simulink model "LATC_Test_Calc"  (R2021b)
settings: Solver=FixedStepDiscrete  StartTime=0.0  StopTime=inf  FixedStep=0.01  RelTol=1e-3
values from neighbouring files (symbols this model uses):
  P_Global_CharSpd_ms : value not decoded    [PubParsGlobal.sldd]
  P_Global_SteeringAngleRatio : value not decoded    [PubParsGlobal.sldd]
  P_Global_WheelBase_m : value not decoded    [PubParsGlobal.sldd]
  P_LCS_A0_Dis_BP : value not decoded    [SubMdlDD_LATC.sldd]
  P_LCS_A2_Curve_BP : value not decoded    [SubMdlDD_LATC.sldd]
  P_LCS_A2_LatAcc_BP : value not decoded    [SubMdlDD_LATC.sldd]
  P_LCS_A2_Pretime = 0.075    [SubMdlDD_LATC.sldd]
  P_LCS_A2S_FliterTime = 0.5    [SubMdlDD_LATC.sldd]
  P_LCS_AngleFilterTime = 0.1    [SubMdlDD_LATC.sldd]
  P_LCS_AngleSlope_AES_Active = 0.4 0.4 0.4 0.35 0.35 0.35 0.35 0.35 0.35 0.3 0.3 0.3 0.3 0.3 0.3 0.3 0.3 0.3 0.3 0.4 0.4 0.4 0.35 0.35 0.35 0.35 0.35 0.35 0.3 0.3 0.3 0.3 0.3 0.3 0.3 0.3 0.3 0.3 0.4 0.4 0.4 0.35 0.35 0.35 0.35 0.35 0.35 0.3 0.3 0.3 0.3 0.3 0.3 0.3 0.3 0.3 0.3 0.4 0.4 0.4 0.35 0.35 0.35 0.35 0.35 0.35 0.3 0.3 0.3 0.3 0.3 0.3 0.3 0.3 0.3 0.3 0.4 0.4 0.4 0.35 0.35 0.35 0.35 0.35 0.35 0.3 0.3 0.3 0.3 0.3 0.3 0.3 0.    [SubMdlDD_LATC.sldd]
  P_LCS_AngleSlope_ESS_Add = 1.0 1.0 1.0 1.0 2.0 2.0 2.0 7.0 7.0 7.0 7.0 7.0 7.0 7.0 7.0 7.0 7.0 7.0 7.0 1.0 1.0 1.0 1.0 2.0 2.0 2.0 7.0 7.0 7.0 7.0 7.0 7.0 7.0 7.0 7.0 7.0 7.0 7.0 1.0 1.0 1.0 1.0 2.0 2.0 2.0 7.0 7.0 7.0 7.0 7.0 7.0 7.0 7.0 7.0 7.0 7.0 7.0 1.0 1.0 1.0 1.0 2.0 2.0 2.0 7.0 7.0 7.0 7.0 7.0 7.0 7.0 7.0 7.0 7.0 7.0 7.0 1.0 1.0 1.0 1.0 7.5 7.5 7.5 7.5 7.5 7.5 7.5 7.5 7.5 7.5 7.5 8.0 8.0 8.0 8.0 1.0 1.0 1.0 1.0 7.5    [SubMdlDD_LATC.sldd]
  P_LCS_AngleSlope_LC_Eco = 0.4 0.4 0.4 0.35 0.35 0.35 0.35 0.35 0.35 0.3 0.3 0.3 0.3 0.3 0.3 0.3 0.3 0.3 0.3 0.4 0.4 0.4 0.35 0.35 0.35 0.35 0.35 0.35 0.3 0.3 0.3 0.3 0.3 0.3 0.3 0.3 0.3 0.3 0.4 0.4 0.4 0.35 0.35 0.35 0.35 0.35 0.35 0.3 0.3 0.3 0.3 0.3 0.3 0.3 0.3 0.3 0.3 0.4 0.4 0.4 0.35 0.35 0.35 0.35 0.35 0.35 0.3 0.3 0.3 0.3 0.3 0.3 0.3 0.3 0.3 0.3 0.4 0.4 0.4 0.35 0.35 0.35 0.35 0.35 0.35 0.3 0.3 0.3 0.3 0.3 0.3 0.3 0.    [SubMdlDD_LATC.sldd]
  P_LCS_AngleSlope_LC_Nomal = 0.4 0.4 0.4 0.35 0.35 0.35 0.35 0.35 0.35 0.3 0.3 0.3 0.3 0.3 0.3 0.3 0.3 0.3 0.3 0.4 0.4 0.4 0.35 0.35 0.35 0.35 0.35 0.35 0.3 0.3 0.3 0.3 0.3 0.3 0.3 0.3 0.3 0.3 0.4 0.4 0.4 0.35 0.35 0.35 0.35 0.35 0.35 0.3 0.3 0.3 0.3 0.3 0.3 0.3 0.3 0.3 0.3 0.4 0.4 0.4 0.35 0.35 0.35 0.35 0.35 0.35 0.3 0.3 0.3 0.3 0.3 0.3 0.3 0.3 0.3 0.3 0.4 0.4 0.4 0.35 0.35 0.35 0.35 0.35 0.35 0.3 0.3 0.3 0.3 0.3 0.3 0.3 0.    [SubMdlDD_LATC.sldd]
  P_LCS_AngleSlope_LC_Sport = 0.4 0.4 0.4 0.35 0.35 0.35 0.35 0.35 0.35 0.3 0.3 0.3 0.3 0.3 0.3 0.3 0.3 0.3 0.3 0.4 0.4 0.4 0.35 0.35 0.35 0.35 0.35 0.35 0.3 0.3 0.3 0.3 0.3 0.3 0.3 0.3 0.3 0.3 0.4 0.4 0.4 0.35 0.35 0.35 0.35 0.35 0.35 0.3 0.3 0.3 0.3 0.3 0.3 0.3 0.3 0.3 0.3 0.4 0.4 0.4 0.35 0.35 0.35 0.35 0.35 0.35 0.3 0.3 0.3 0.3 0.3 0.3 0.3 0.3 0.3 0.3 0.4 0.4 0.4 0.35 0.35 0.35 0.35 0.35 0.35 0.3 0.3 0.3 0.3 0.3 0.3 0.3 0.    [SubMdlDD_LATC.sldd]
  P_LCS_AngleSlope_LCK = 0.4 0.4 0.4 0.4 0.4 0.4 0.4 0.4 0.4 0.4 0.4 0.4 0.4 0.4 0.4 0.4 0.4 0.4 0.4 0.4 0.4 0.4 0.4 0.4 0.4 0.4 0.4 0.4 0.4 0.4 0.4 0.4 0.4 0.4 0.4 0.4 0.4 0.4 0.4 0.4 0.4 0.4 0.4 0.4 0.4 0.4 0.4 0.4 0.4 0.4 0.4 0.4 0.4 0.4 0.4 0.4 0.4 0.4 0.4 0.4 0.4 0.4 0.4 0.4 0.4 0.4 0.4 0.4 0.4 0.4 0.4 0.4 0.4 0.4 0.4 0.4 0.4 0.4 0.4 0.4 0.4 0.4 0.4 0.4 0.4 0.4 0.4 0.4 0.4 0.4 0.4 0.4 0.4 0.4 0.4 0.4 0.4 0.4 0.4 0.4    [SubMdlDD_LATC.sldd]
  P_LCS_AngleSlope_LCKIE = 0.4 0.4 0.4 0.4 0.4 0.4 0.4 0.4 0.4 0.4 0.4 0.4 0.4 0.4 0.4 0.4 0.4 0.4 0.4 0.4 0.4 0.4 0.4 0.4 0.4 0.4 0.4 0.4 0.4 0.4 0.4 0.4 0.4 0.4 0.4 0.4 0.4 0.4 0.4 0.4 0.4 0.4 0.4 0.4 0.4 0.4 0.4 0.4 0.4 0.4 0.4 0.4 0.4 0.4 0.4 0.4 0.4 0.4 0.4 0.4 0.4 0.4 0.4 0.4 0.4 0.4 0.4 0.4 0.4 0.4 0.4 0.4 0.4 0.4 0.4 0.4 0.4 0.4 0.4 0.4 0.4 0.4 0.4 0.4 0.4 0.4 0.4 0.4 0.4 0.4 0.4 0.4 0.4 0.4 0.4 0.4 0.4 0.4 0.4 0.4    [SubMdlDD_LATC.sldd]
  P_LCS_AngleSlope_LKA = 0.2 0.2 0.3 0.4 0.4 0.4 0.4 0.4 0.4 0.4 0.4 0.4 0.4 0.4 0.4 0.4 0.4 0.4 0.4 0.2 0.2 0.3 0.4 0.4 0.4 0.4 0.4 0.4 0.4 0.4 0.4 0.4 0.4 0.4 0.4 0.4 0.4 0.4 0.2 0.2 0.3 0.4 0.4 0.4 0.4 0.4 0.4 0.4 0.4 0.4 0.4 0.4 0.4 0.4 0.4 0.4 0.4 0.2 0.2 0.3 0.4 0.4 0.4 0.4 0.4 0.4 0.4 0.4 0.4 0.4 0.4 0.4 0.4 0.4 0.4 0.4 0.2 0.2 0.3 0.4 0.4 0.4 0.4 0.4 0.4 0.4 0.4 0.4 0.4 0.4 0.4 0.4 0.4 0.4 0.4 0.2 0.2 0.3 0.4 0.4    [SubMdlDD_LATC.sldd]
  P_LCS_AngleSlope_Spd_BP : value not decoded    [SubMdlDD_LATC.sldd]
  P_LCS_DeltaEps_SpdBp : value not decoded    [SubMdlDD_LATC.sldd]
  P_LCS_DeltaEps_TimeVal : value not decoded    [SubMdlDD_LATC.sldd]
  P_LCS_DetNoOverRide_DrvTrq_TH : value not decoded    [SubMdlDD_LATC.sldd]
  P_LCS_DetOverRide_DrvTrq_TH : value not decoded    [SubMdlDD_LATC.sldd]
  P_LCS_ESS_AngleSlope_Limit = 2.9    [SubMdlDD_LATC.sldd]
  P_LCS_ESSAngleSW2 = 0.0    [SubMdlDD_LATC.sldd]
  P_LCS_LatAcc2CurveSW = 0.0    [SubMdlDD_LATC.sldd]
  P_LCS_LC_Complete_PreDisFac : value not decoded    [SubMdlDD_LATC.sldd]
  P_LCS_LCK_preDis_Nomal : value not decoded    [SubMdlDD_LATC.sldd]
  P_LCS_NoOverRideTime_TH_s : value not decoded    [SubMdlDD_LATC.sldd]
  P_LCS_OverRideDetect_enable : value not decoded    [SubMdlDD_LATC.sldd]
  P_LCS_OverRideTime_TH_s : value not decoded    [SubMdlDD_LATC.sldd]
  P_LCS_preDis_AES_Fac = 0.0 0.0 0.0 0.0 -0.1 -0.1 -0.1 -0.1 -0.1 -0.1 0.1 0.1 0.1 0.2 0.2 0.2 0.2 0.2 0.2 0.0 0.0 0.0 0.0 -0.1 -0.1 -0.1 -0.1 -0.1 -0.1 0.1 0.1 0.1 0.2 0.2 0.2 0.2 0.2 0.2 0.0 0.0 0.0 0.0 -0.1 -0.1 -0.1 -0.1 -0.1 -0.1 0.1 0.1 0.1 0.2 0.2 0.2 0.2 0.2 0.2 0.0 0.0 0.0 0.0 -0.1 -0.1 -0.1 -0.1 -0.1 -0.1 0.1 0.1 0.1 0.2 0.2 0.2 0.2 0.2 0.2 0.0 0.0 0.0 0.0 -0.1 -0.1 -0.1 -0.1 -0.1 -0.1 0.2 0.2 0.2 0.35 0.35 0.35    [SubMdlDD_LATC.sldd]
  P_LCS_preDis_LC_Eco_Fac = 0.0 0.0 0.0 0.0 0.25 0.3 0.3 0.3 0.35 0.35 0.45 0.45 0.45 0.55 0.55 0.55 0.55 0.55 0.55 0.0 0.0 0.0 0.0 0.25 0.3 0.3 0.3 0.35 0.35 0.45 0.45 0.45 0.55 0.55 0.55 0.55 0.55 0.55 0.0 0.0 0.0 0.0 0.25 0.3 0.3 0.3 0.35 0.35 0.45 0.45 0.45 0.55 0.55 0.55 0.55 0.55 0.55 0.0 0.0 0.0 0.0 0.25 0.3 0.3 0.3 0.35 0.35 0.45 0.45 0.45 0.55 0.55 0.55 0.55 0.55 0.55 0.0 0.0 0.0 0.0 0.25 0.3 0.3 0.3 0.35 0.35 0.55    [SubMdlDD_LATC.sldd]
  P_LCS_preDis_LC_Fac = 0.0 0.0 0.0 0.0 -0.1 -0.1 -0.1 -0.1 -0.1 -0.1 0.1 0.1 0.1 0.2 0.2 0.2 0.2 0.2 0.2 0.0 0.0 0.0 0.0 -0.1 -0.1 -0.1 -0.1 -0.1 -0.1 0.1 0.1 0.1 0.2 0.2 0.2 0.2 0.2 0.2 0.0 0.0 0.0 0.0 -0.1 -0.1 -0.1 -0.1 -0.1 -0.1 0.1 0.1 0.1 0.2 0.2 0.2 0.2 0.2 0.2 0.0 0.0 0.0 0.0 -0.1 -0.1 -0.1 -0.1 -0.1 -0.1 0.1 0.1 0.1 0.2 0.2 0.2 0.2 0.2 0.2 0.0 0.0 0.0 0.0 -0.1 -0.1 -0.1 -0.1 -0.1 -0.1 0.2 0.2 0.2 0.35 0.35 0.35    [SubMdlDD_LATC.sldd]
  P_LCS_preDis_LC_Nomal_Fac = 0.0 0.0 0.0 0.0 -0.1 -0.1 -0.1 -0.1 -0.1 -0.1 0.1 0.1 0.1 0.2 0.2 0.2 0.2 0.2 0.2 0.0 0.0 0.0 0.0 -0.1 -0.1 -0.1 -0.1 -0.1 -0.1 0.1 0.1 0.1 0.2 0.2 0.2 0.2 0.2 0.2 0.0 0.0 0.0 0.0 -0.1 -0.1 -0.1 -0.1 -0.1 -0.1 0.1 0.1 0.1 0.2 0.2 0.2 0.2 0.2 0.2 0.0 0.0 0.0 0.0 -0.1 -0.1 -0.1 -0.1 -0.1 -0.1 0.1 0.1 0.1 0.2 0.2 0.2 0.2 0.2 0.2 0.0 0.0 0.0 0.0 -0.1 -0.1 -0.1 -0.1 -0.1 -0.1 0.2 0.2 0.2 0.35 0.35 0.35    [SubMdlDD_LATC.sldd]
  P_LCS_preDis_LC_Sport_Fac = 0.0 0.0 0.0 0.0 -0.1 -0.1 -0.1 -0.1 -0.1 -0.1 0.1 0.1 0.1 0.2 0.2 0.2 0.2 0.2 0.2 0.0 0.0 0.0 0.0 -0.1 -0.1 -0.1 -0.1 -0.1 -0.1 0.1 0.1 0.1 0.2 0.2 0.2 0.2 0.2 0.2 0.0 0.0 0.0 0.0 -0.1 -0.1 -0.1 -0.1 -0.1 -0.1 0.1 0.1 0.1 0.2 0.2 0.2 0.2 0.2 0.2 0.0 0.0 0.0 0.0 -0.1 -0.1 -0.1 -0.1 -0.1 -0.1 0.1 0.1 0.1 0.2 0.2 0.2 0.2 0.2 0.2 0.0 0.0 0.0 0.0 -0.1 -0.1 -0.1 -0.1 -0.1 -0.1 0.2 0.2 0.2 0.35 0.35 0.35    [SubMdlDD_LATC.sldd]
  P_LCS_preDis_LCK_A2Curve_Fac2 : value not decoded    [SubMdlDD_LATC.sldd]
  P_LCS_preDis_spd : value not decoded    [SubMdlDD_LATC.sldd]
  P_LCS_StateActive_HoldTime_BP : value not decoded    [SubMdlDD_LATC.sldd]
  P_LCS_StateComplete_AngleSlope : value not decoded    [SubMdlDD_LATC.sldd]
  P_LCS_StateCompleteFlg_BP : value not decoded    [SubMdlDD_LATC.sldd]
  P_LCS_StateHold_time = 250.0    [SubMdlDD_LATC.sldd]
undefined symbols (not defined in the file or in its folder): P_LCS_AngleSlope_ELK, P_LCS_AngleSlope_ESS, P_LCS_AngleSlope_LC_Cancel, P_LCS_AngleSlope_LCK_Curve_Fac, P_LCS_ESS_preDis_Nomal, P_LCS_ESSAngleSW, P_LCS_ESSAngSlope_SW, P_LCS_preDis_ELK_Fac, P_LCS_preDis_ESS_Fac, P_LCS_preDis_LCK_A2Curve_Fac, P_LCS_preDis_LCK_Fac, P_LCS_StateActiv_AngleSlope, P_LCS_StateActiveFlg_BP
libraries: canapelib x26, simulink x7
(part 1 of 2)
settings Model: DataDictionary=SubMdlDD_LATC.sldd  Creator=GW00216231  LastModifiedBy=GW00216231
settings SolverCC: AlgebraicLoopSolver=TrustRegion
settings OptimizationCC: DefaultParameterBehavior=Inlined  EnhancedBackFolding=on  PassReuseOutputArgsThreshold=0  OptimizeBlockOrder=speed  DifferentSizesBufferReuse=on  OptimizationCustomize=off
settings DebuggingCC: SignalResolutionControl=TryResolveAllWithWarning  ParameterTunabilityLossMsg=error  SFMachineParentedDataDiag=warning  UnderSpecifiedDimensionMsg=warning
settings SFSimCC: MATLABDynamicMemAlloc=off
settings RTWCC: Description=Vector CANape/vSignalyzer Target (Visual C/C++ Project Makefile)  SystemTargetFile=cnp.tlc  TemplateMakefile=cnp_msdll.tmf
settings CodeAppCC: ForceParamTrailComments=on  OperatorAnnotations=on
settings STFCustomTargetCC: TargetLangStandard=C99 (ISO)  MATLABClassNameForMDSCustomization=Simulink.SoftwareTarget.TargetSpecificTriggerConfigurationBase  SystemTargetFile=cnp.tlc

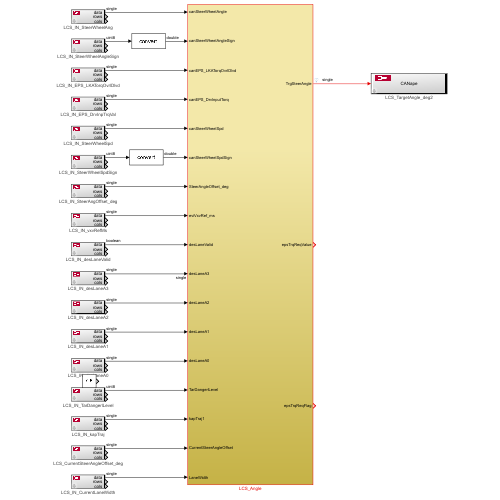
[thumbnail: Simulink's stored preview of the top-level diagram]
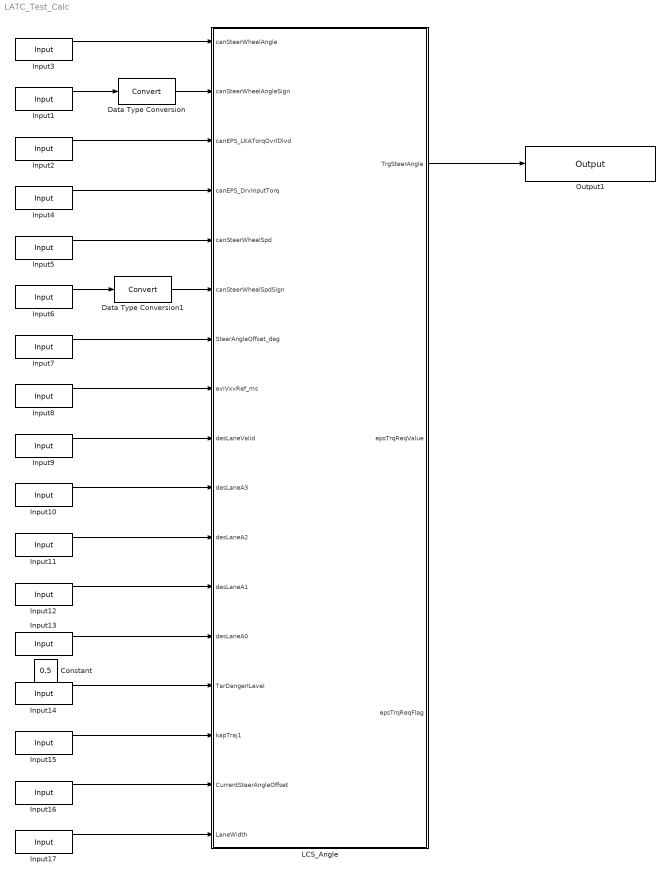
== system LATC_Test_Calc ==
  Constant : Constant  Value=0.5  OutDataTypeStr=single
  Data Type Conversion : DataTypeConversion
  Data Type Conversion1 : DataTypeConversion
  Input1 : canapelib/CANape I//O/Input  envName=LCS_IN_SteerWheelAngleSign  envRows=1  envCols=1  envDataType=uint8  swInheritSampleTime=on  envPortId=0
      settings: AttributesFormatString=%<envName>  SourceProductName=Vector CANape/vSignalyzer Target
  Input10 : canapelib/CANape I//O/Input  envName=LCS_IN_desLaneA3  envRows=1  envCols=1  envDataType=float  swInheritSampleTime=on  envPortId=0
      settings: AttributesFormatString=%<envName>  SourceProductName=Vector CANape/vSignalyzer Target
  Input11 : canapelib/CANape I//O/Input  envName=LCS_IN_desLaneA2  envRows=1  envCols=1  envDataType=float  swInheritSampleTime=on  envPortId=0
      settings: AttributesFormatString=%<envName>  SourceProductName=Vector CANape/vSignalyzer Target
  Input12 : canapelib/CANape I//O/Input  envName=LCS_IN_desLaneA1  envRows=1  envCols=1  envDataType=float  swInheritSampleTime=on  envPortId=0
      settings: AttributesFormatString=%<envName>  SourceProductName=Vector CANape/vSignalyzer Target
  Input13 : canapelib/CANape I//O/Input  envName=LCS_IN_desLaneA0  envRows=1  envCols=1  envDataType=float  swInheritSampleTime=on  envPortId=0
      settings: AttributesFormatString=%<envName>  SourceProductName=Vector CANape/vSignalyzer Target
  Input14 : canapelib/CANape I//O/Input  envName=LCS_IN_TarDangerlLevel  envRows=1  envCols=1  envDataType=uint8  swInheritSampleTime=on  envPortId=0
      settings: AttributesFormatString=%<envName>  SourceProductName=Vector CANape/vSignalyzer Target
  Input15 : canapelib/CANape I//O/Input  envName=LCS_IN_kapTraj  envRows=1  envCols=1  envDataType=float  swInheritSampleTime=on  envPortId=0
      settings: AttributesFormatString=%<envName>  SourceProductName=Vector CANape/vSignalyzer Target
  Input16 : canapelib/CANape I//O/Input  envName=LCS_CurrentSteerAngleOffset_deg  envRows=1  envCols=1  envDataType=float  swInheritSampleTime=on  envPortId=0
      settings: AttributesFormatString=%<envName>  SourceProductName=Vector CANape/vSignalyzer Target
  Input17 : canapelib/CANape I//O/Input  envName=LCS_IN_CurrentLaneWidth  envRows=1  envCols=1  envDataType=float  swInheritSampleTime=on  envPortId=0
      settings: AttributesFormatString=%<envName>  SourceProductName=Vector CANape/vSignalyzer Target
  Input2 : canapelib/CANape I//O/Input  envName=LCS_IN_EPS_LKATorqOvrlDlvd  envRows=1  envCols=1  envDataType=float  swInheritSampleTime=on  envPortId=0
      settings: AttributesFormatString=%<envName>  SourceProductName=Vector CANape/vSignalyzer Target
  Input3 : canapelib/CANape I//O/Input  envName=LCS_IN_SteerWheelAng  envRows=1  envCols=1  envDataType=float  swInheritSampleTime=on  envPortId=0
      settings: AttributesFormatString=%<envName>  SourceProductName=Vector CANape/vSignalyzer Target
  Input4 : canapelib/CANape I//O/Input  envName=LCS_IN_EPS_DrvInpTrqVal  envRows=1  envCols=1  envDataType=float  swInheritSampleTime=on  envPortId=0
      settings: AttributesFormatString=%<envName>  SourceProductName=Vector CANape/vSignalyzer Target
  Input5 : canapelib/CANape I//O/Input  envName=LCS_IN_SteerWheelSpd  envRows=1  envCols=1  envDataType=float  swInheritSampleTime=on  envPortId=0
      settings: AttributesFormatString=%<envName>  SourceProductName=Vector CANape/vSignalyzer Target
  Input6 : canapelib/CANape I//O/Input  envName=LCS_IN_SteerWheelSpdSign  envRows=1  envCols=1  envDataType=uint8  swInheritSampleTime=on  envPortId=0
      settings: AttributesFormatString=%<envName>  SourceProductName=Vector CANape/vSignalyzer Target
  Input7 : canapelib/CANape I//O/Input  envName=LCS_IN_SteerAngOffset_deg  envRows=1  envCols=1  envDataType=float  swInheritSampleTime=on  envPortId=0
      settings: AttributesFormatString=%<envName>  SourceProductName=Vector CANape/vSignalyzer Target
  Input8 : canapelib/CANape I//O/Input  envName=LCS_IN_vxvRefMs  envRows=1  envCols=1  envDataType=float  swInheritSampleTime=on  envPortId=0
      settings: AttributesFormatString=%<envName>  SourceProductName=Vector CANape/vSignalyzer Target
  Input9 : canapelib/CANape I//O/Input  envName=LCS_IN_desLaneValid  envRows=1  envCols=1  envDataType=boolean  swInheritSampleTime=on  envPortId=0
      settings: AttributesFormatString=%<envName>  SourceProductName=Vector CANape/vSignalyzer Target
  LCS_Angle : Subsystem
  Output1 : canapelib/CANape I//O/Output  envName=LCS_TargetAngle_deg2  envRows=1  envCols=1  envPortId=0
      settings: AttributesFormatString=%<envName>  SourceProductName=Vector CANape/vSignalyzer Target
  wires:
  Input3/1 -> LCS_Angle/1(canSteerWheelAngle)
  Input1/1 -> Data Type Conversion/1
  Input2/1 -> LCS_Angle/3(canEPS_LKATorqOvrlDlvd)
  Input4/1 -> LCS_Angle/4(canEPS_DrvInputTorq)
  Input5/1 -> LCS_Angle/5(canSteerWheelSpd)
  Input6/1 -> Data Type Conversion1/1
  Input7/1 -> LCS_Angle/7(SteerAngleOffset_deg)
  Input8/1 -> LCS_Angle/8(eviVxvRef_ms)
  Input9/1 -> LCS_Angle/9(desLaneValid)
  Input10/1 -> LCS_Angle/10(desLaneA3)
  Input11/1 -> LCS_Angle/11(desLaneA2)
  Input12/1 -> LCS_Angle/12(desLaneA1)
  Input13/1 -> LCS_Angle/13(desLaneA0)
  Input14/1 -> LCS_Angle/14(TarDangerlLevel)
  Input15/1 -> LCS_Angle/15(kapTraj1)
  Input16/1 -> LCS_Angle/16(CurrentSteerAngleOffset)
  Input17/1 -> LCS_Angle/17(LaneWidth)
  LCS_Angle/1(TrgSteerAngle) -> Output1/1
  Data Type Conversion/1 -> LCS_Angle/2(canSteerWheelAngleSign)
  Data Type Conversion1/1 -> LCS_Angle/6(canSteerWheelSpdSign)

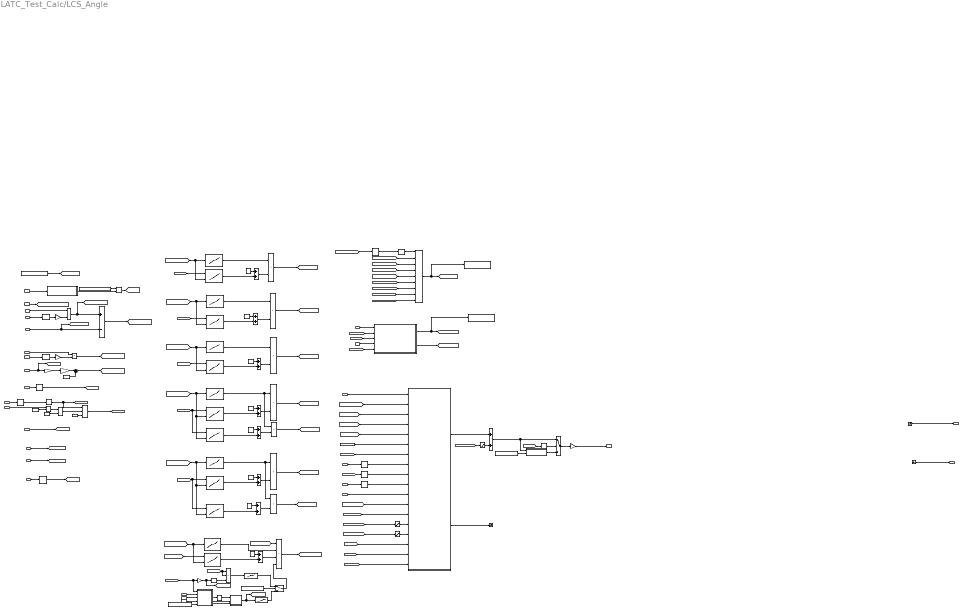
== system LATC_Test_Calc/LCS_Angle ==
  note: 0:No Function Active
      | 1:LCK Active
      | 2:LCKIE Active
      | 3:LC Normal Active
      | 4:LKA Active
      | 5:ELK Active
      | 6:ESS Active
      | 7:LC Eco Active
      | 8:LC Sport Active
      | 9:LC cancel
      | 10: AES Active
  note: ESS_AES
  note: ELK && LC
  note: Steer Wheel Angle Slope Manage
  note: LCK_LKA_LCKIE_Normal
  note: Sport
  note: Eco
  note: Normal
  note: PreDis_Manage
  note: Torque
  note: 模型变更记录
      | 2021/05/31 修改PreDis观测量、增加PreDisFac观测量；（版本：36010506）
      | 2021/06/02 增加弯道关于A2的PreDisFac标定量；（版本：36010506）
      | 2021/06/08 按A0 = 0.8m退出LC修改三种换道预瞄距离系数；增加LCS_EpsTrqReqValue、LCS_EpsTrqReqValueVld观测量（版本：36010506）
      | 2021/06/17 增加单独的ELK、ESSAES预瞄距离参数表；增加LCS_LC_ESSPredis、LCS_LC_ELKPredis观测量；增加ESS、ELS手动调试开关（版本：36170507）
      | 修改LCS模型输出观测量命名，例：LCS_ReqEPSTrgAngle -> LCS_OUT_ReqEPSTrgAngle
      | 2021/07/05 更新ELK标定参数（版本：37050508）
      | 2021/07/12 更新P_LCS_preDis_LCK_A2Curve_Fac标定参数（版本：37120509）
      | 2021/07/15 增加弯道内通过预瞄曲率查表LCK_Predis的Fac修正系数逻辑（版本：37120509）
      | 2021/07/20 增加换道取消P_LCS_preDis_LC_Fac修正系数（版本：37120509）
      | 2021/08/03 增加ESS请求角度斜率限制，防止EPS故障（版本：37120509）
      | 2021/08/04 增加EPS转速>150，ESS退出逻辑，暂用于测试，后期可能会删除（版本：37120509）
      | 2021/08/04 P_LCS_LatAcc2CurveSW设置默认为0
      | 2021/08/09 增加ESS测试逻辑，暂时测试版
      | 2021/08/16 ESS标定数据更改、增加转角与扭矩得ESS开关
      | 2021/08/20 A2项逻辑默认开，LCK_Fac全部置0，P_LCS_preDis_LCK_A2Curve_Fac2参数置：1 1 1 0.85 0.75 0.6 0.5 0.3 0.3 0.25
      | 2021/08/21 修改5kph以下LineValid置零逻辑（版本：38210511）
      | 2021/08/23 修改5kph以下LineValid置零，置零后目标角度不滤波（版本：38210511）
      | 2021/08/23 修改LC换道取消逻辑和标定参数（版本：38230512）
      | 2021/08/24 ESS最初为~=6，因测试出当DangerLevel==6时，状态可能跳变的问题。改成<=5，避免数据类型导致数据比较出现的问题
      | 2021/08/24 增加EPS故障监控逻辑、PID中FF和Kp增加A0项（版本：38240513）
      | 2021/08/25 修改AngleErrorRevers反向符号逻辑（版本：38250514）
      | 2021/08/30 模型整理（版本：38300515）
      | 2021/09/07 修改ESS置位条件（版本：39070516）
      | 2021/09/15 增加port口描述及接口数据类型（版本：39150517）
      | 2021/10/18 LineValid置零逻辑阈值由5kph->3kph;同步CurrentOffset激活逻辑;增加换道超调控制逻辑(默认关闭)（版本：10180518）
      | 2021/10/20 修改内部CurrentOffset激活条件，改成根据曲率进行滤波（版本：10200519)
      | 2021/11/01 增加大框接口LATC_Effect（版本：11010520)
      | 2021/11/03 增加依据曲率修正LCK的AngelSlope（版本：11030521)
      | 2021/11/04 增加内部CurrentOffset计算限值（版本：11040522)
      | 2021/11/08 修改内部CurrentOffset根据曲率进行滤波的时间（版本：11080523)
  note: ESS请求角度斜率限制，防止EPS故障
  canSteerWheelAngle : Inport
  canSteerWheelAngleSign : Inport  Port=2
  canEPS_LKATorqOvrlDlvd : Inport  Port=3
  canEPS_DrvInputTorq : Inport  Port=4
  canSteerWheelSpd : Inport  Port=5
  canSteerWheelSpdSign : Inport  Port=6
  SteerAngleOffset_deg : Inport  Port=7
  eviVxvRef_ms : Inport  Port=8
  desLaneValid : Inport  Port=9
  desLaneA3 : Inport  Port=10  OutDataTypeStr=single
  desLaneA2 : Inport  Port=11
  desLaneA1 : Inport  Port=12
  desLaneA0 : Inport  Port=13
  TarDangerlLevel : Inport  Port=14
  kapTraj1 : Inport  Port=15
  CurrentSteerAngleOffset : Inport  Port=16
  LaneWidth : Inport  Port=17
  2-D Lookup Table1 : Lookup_n-D  BreakpointsForDimension1=P_LCS_A0_Dis_BP  BreakpointsForDimension2=P_LCS_preDis_spd  Table=P_LCS_preDis_LC_Nomal_Fac  ExtrapMethod=Clip  UseLastTableValue=on  InternalRulePriority=Speed  RndMeth=Simplest  InputSameDT=on
      settings: InputPortMap=u0,u1
  2-D Lookup Table2 : Lookup_n-D  BreakpointsForDimension1=P_LCS_A0_Dis_BP  BreakpointsForDimension2=P_LCS_preDis_spd  Table=P_LCS_preDis_LCK_Fac  ExtrapMethod=Clip  UseLastTableValue=on  InternalRulePriority=Speed  RndMeth=Simplest  InputSameDT=on
      settings: InputPortMap=u0,u1
  Abs1 : Abs
  Abs2 : Abs
  Abs4 : Abs
  Add1 : Sum  Inputs=+-
  Add{2,5,7..12} (8 alike) : Sum
  Add6 : Sum  AccumDataTypeStr=single
  AngSlopeCalc : Subsystem
  Bias1 : Bias  Bias=-0.5
  Bias2 : Bias  Bias=-0.5
  Compare To Constant1 : simulink/Logic and Bit Operations/Compare To Constant  relop=~=  const=6  OutDataTypeStr=boolean
  Constant : Constant  Value=P_Global_SteeringAngleRatio  OutDataTypeStr=double
  Constant1 : Constant  Value=1000  OutDataTypeStr=single
  Constant{12..14,17..18,22,24,26} (8 alike) : Constant  OutDataTypeStr=single
  Constant15 : Constant  Value=P_LCS_OverRideDetect_enable
  Constant16 : Constant  Value=P_LCS_ESS_AngleSlope_Limit  OutDataTypeStr=single
  Constant2 : Constant  Value=P_LCS_LatAcc2CurveSW
  Constant20 : Constant  Value=P_LCS_A2S_FliterTime
  Constant21 : Constant  Value=P_LCS_A2_Pretime  OutDataTypeStr=single
  Constant4 : Constant  Value=3.6  OutDataTypeStr=single
  Constant6 : Constant  Value=3  OutDataTypeStr=single
  Constant7 : Constant  Value=4  OutDataTypeStr=single
  Constant8 : Constant  Value=1.3  OutDataTypeStr=single
  Direct Lookup Table (n-D) : LookupNDDirect  NumberOfTableDimensions=1  Table=[4 4 4 1 4 5 6 2 3 7 8]  TableDataTypeStr=uint8
  Divide : Product  Inputs=**/
  Gain : Gain  Gain=-1
  Gain1 : Gain  Gain=2
  Gain2 : Gain  Gain=-2  OutDataTypeStr=single
  Gain3 : Gain  Gain=3.6
  Gain4 : Gain  Gain=1.03
  Gain5 : Gain  Gain=-2  OutDataTypeStr=single
  Ground : Ground
  Ground1 : Ground
  LCS_LC_ELK_preDis_TB : Lookup_n-D  BreakpointsForDimension1=P_LCS_A0_Dis_BP  BreakpointsForDimension2=P_LCS_preDis_spd  Table=P_LCS_preDis_ELK_Fac  ExtrapMethod=Clip  UseLastTableValue=on  InternalRulePriority=Speed  RndMeth=Simplest  InputSameDT=on
      settings: InputPortMap=u0,u1
  LCS_LC_ELK_preDis_TB1 : Lookup_n-D  BreakpointsForDimension1=P_LCS_A0_Dis_BP  BreakpointsForDimension2=P_LCS_preDis_spd  Table=P_LCS_preDis_LC_Fac  ExtrapMethod=Clip  UseLastTableValue=on  InternalRulePriority=Speed  RndMeth=Simplest  InputSameDT=on
      settings: InputPortMap=u0,u1
  LCS_LC_ESSAES_preDis_TB : Lookup_n-D  BreakpointsForDimension1=P_LCS_A0_Dis_BP  BreakpointsForDimension2=P_LCS_preDis_spd  Table=P_LCS_preDis_ESS_Fac  ExtrapMethod=Clip  UseLastTableValue=on  InternalRulePriority=Speed  RndMeth=Simplest  InputSameDT=on
      settings: InputPortMap=u0,u1
  LCS_LC_ESSAES_preDis_TB1 : Lookup_n-D  BreakpointsForDimension1=P_LCS_A0_Dis_BP  BreakpointsForDimension2=P_LCS_preDis_spd  Table=P_LCS_preDis_AES_Fac  ExtrapMethod=Clip  UseLastTableValue=on  InternalRulePriority=Speed  RndMeth=Simplest  InputSameDT=on
      settings: InputPortMap=u0,u1
  LCS_LC_Emergent_preDis_TB : Lookup_n-D  BreakpointsForDimension1=P_LCS_A0_Dis_BP  BreakpointsForDimension2=P_LCS_preDis_spd  Table=P_LCS_preDis_LC_Sport_Fac  ExtrapMethod=Clip  UseLastTableValue=on  InternalRulePriority=Speed  RndMeth=Simplest  InputSameDT=on
      settings: InputPortMap=u0,u1
  LC_Medium_preDis_Fac_TB : Lookup_n-D  BreakpointsForDimension1=P_LCS_A0_Dis_BP  BreakpointsForDimension2=P_LCS_preDis_spd  Table=P_LCS_preDis_LC_Eco_Fac  ExtrapMethod=Clip  UseLastTableValue=on  InternalRulePriority=Speed  RndMeth=Simplest  InputSameDT=on
      settings: InputPortMap=u0,u1
  LP filter : Subsystem
  Logical Operator1 : Logic  AllPortsSameDT=off  OutDataTypeStr=boolean
  MATLAB Function : MATLAB Function  TreatAsAtomicUnit=on
  MinMax : MinMax  Function=max  Inputs=2
  MinMax1 : MinMax  Inputs=2
  Multiport Switch4 : MultiPortSwitch  Inputs=8
  Output1 : canapelib/CANape I//O/Output  envName=LCS_TarSteerAngleSlope2  envRows=1  envCols=1  envPortId=0
      settings: AttributesFormatString=%<envName>  SourceProductName=Vector CANape/vSignalyzer Target
  Output2 : canapelib/CANape I//O/Output  envName=LCS_finalPredis2  envRows=1  envCols=1  envPortId=0
      settings: AttributesFormatString=%<envName>  SourceProductName=Vector CANape/vSignalyzer Target
  OverRideDetect : Subsystem
  Product1 : Product  Inputs=3
  Product{3..9,12,15} (9 alike) : Product
  Product2 : Product  Inputs=4
  Saturation : Saturate  UpperLimit=10  LowerLimit=-10
  Saturation1 : Saturate  UpperLimit=10  LowerLimit=-10
  Saturation2 : Saturate  UpperLimit=10  LowerLimit=-10
  Signal Copy{,1..6} (7 alike) : SignalConversion  OverrideOpt=off
  Subsystem5 : Subsystem
  Sum : Sum  Inputs=|++
  Switch : Switch  Criteria=u2 ~= 0
  Switch1 : Switch  Criteria=u2 > Threshold
  TarDangerlLevel2 : InportShadow  Port=14
  TargetSteerAngleCalc : Subsystem
  Terminator : Terminator
  desLaneA0_1 : InportShadow  Port=13
  desLaneA0_2 : InportShadow  Port=13
  desLaneA1_4 : InportShadow  Port=12
  desLaneA3_4 : InportShadow  Port=10  OutDataTypeStr=single
  eviVxvRef_ms1 : InportShadow  Port=8
  eviVxvRef_ms6 : InportShadow  Port=8
  preDisMin_TB : Lookup_n-D  NumberOfTableDimensions=1  BreakpointsForDimension1=P_LCS_preDis_spd  Table=P_LCS_LCK_preDis_Nomal  ExtrapMethod=Clip  InternalRulePriority=Speed  RndMeth=Simplest  InputSameDT=on
  preDisMin_TB1 : Lookup_n-D  NumberOfTableDimensions=1  BreakpointsForDimension1=P_LCS_preDis_spd  Table=P_LCS_LCK_preDis_Nomal  ExtrapMethod=Clip  InternalRulePriority=Speed  RndMeth=Simplest  InputSameDT=on
  preDisMin_TB2 : Lookup_n-D  NumberOfTableDimensions=1  BreakpointsForDimension1=P_LCS_preDis_spd  Table=P_LCS_LCK_preDis_Nomal  ExtrapMethod=Clip  UseLastTableValue=on  InternalRulePriority=Speed  RndMeth=Simplest  InputSameDT=on
  preDisMin_TB3 : Lookup_n-D  NumberOfTableDimensions=1  BreakpointsForDimension1=P_LCS_preDis_spd  Table=P_LCS_LCK_preDis_Nomal  ExtrapMethod=Clip  UseLastTableValue=on  InternalRulePriority=Speed  RndMeth=Simplest  InputSameDT=on
  preDisMin_TB4 : Lookup_n-D  NumberOfTableDimensions=1  BreakpointsForDimension1=P_LCS_preDis_spd  Table=P_LCS_LCK_preDis_Nomal  ExtrapMethod=Clip  InternalRulePriority=Speed  RndMeth=Simplest  InputSameDT=on
  preDisMin_TB5 : Lookup_n-D  NumberOfTableDimensions=1  BreakpointsForDimension1=P_LCS_preDis_spd  Table=P_LCS_ESS_preDis_Nomal  ExtrapMethod=Clip  InternalRulePriority=Speed  RndMeth=Simplest  InputSameDT=on
  predis_ayFac1 : Lookup_n-D  NumberOfTableDimensions=1  BreakpointsForDimension1=P_LCS_A2_Curve_BP  Table=P_LCS_preDis_LCK_A2Curve_Fac2  ExtrapMethod=Clip  UseLastTableValue=on  InternalRulePriority=Speed  RndMeth=Simplest  InputSameDT=on
  predis_ayFac4 : Lookup_n-D  NumberOfTableDimensions=1  BreakpointsForDimension1=P_LCS_A2_LatAcc_BP  Table=P_LCS_preDis_LCK_A2Curve_Fac  ExtrapMethod=Clip  UseLastTableValue=on  InternalRulePriority=Speed  RndMeth=Simplest  InputSameDT=on
  TrgSteerAngle : Outport  OutDataTypeStr=single
  epsTrqReqValue : Outport  Port=2
  epsTrqReqFlag : Outport  Port=3
  wires:
  [Predis_Curve] -> AngSlopeCalc/5(Predis_Curve)
  [LC_Complete_PreDisFac] -> Product2/1
  Signal Copy6/1 -> [TarDangerlLevel]  "LCS_IN_TarDangerlLevel"
  [TarDangerlLevel] -> Signal Copy/1
  [DisplaySpd_kph] -> TargetSteerAngleCalc/18(DisplaySpd_kph)
  [Eq_A0] -> TargetSteerAngleCalc/17(Eq_A0)
  [AES_PreDis] -> Multiport Switch4/9
  Product9/1 -> [AES_PreDis]  "LCS_LC_AESPredis"
  Add12/1 -> Product9/2
  LCS_LC_ESSAES_preDis_TB1/1 -> Add12/2  "LCS_LC_AESPredisFac"
  Constant17/1 -> Add12/1
  [TarDangerlLevel] -> TargetSteerAngleCalc/16(TarDangerlLevel)
  Constant16/1 -> Subsystem5/2(Slope)
  Subsystem5/1(out) -> Switch1/3
  Switch1/1 -> Gain/1
  Compare To Constant1/1 -> Switch1/2
  [TarDangerlLevel] -> Compare To Constant1/1
  AngSlopeCalc/2(LC_Complete_PreDisFac) -> [LC_Complete_PreDisFac]  "LCS_LC_Complete_PreDisFac"
  [LC_PreDis] -> Multiport Switch4/8
  Product8/1 -> [LC_PreDis]  "LCS_LC_LCPredis"
  Add11/1 -> Product8/2
  LCS_LC_ELK_preDis_TB1/1 -> Add11/2  "LCS_LC_LCPredisFac"
  Constant18/1 -> Add11/1
  predis_ayFac1/1 -> Switch/3  "LCS_Predis_CurveFac"
  Switch/1 -> Product2/4  "LCS_LCK_CurveFac"
  LP filter/1(output) -> predis_ayFac1/1, [Predis_Curve]  "LCS_Predis_Curve"
  Constant2/1 -> Switch/2
  Constant20/1 -> LP filter/2(TorqFilterTime)
  Abs4/1 -> LP filter/1(Raw)
  MATLAB Function/1(PreCurve) -> Abs4/1
  Constant21/1 -> MATLAB Function/5(time)
  eviVxvRef_ms1/1 -> MATLAB Function/4(v)
  desLaneA3_4/1 -> MATLAB Function/3(c3)
  desLaneA1_4/1 -> MATLAB Function/2(c1)
  desLaneValid/1 -> Signal Copy4/1
  Signal Copy3/1 -> TargetSteerAngleCalc/10(A1)  "LCS_IN_desLaneA1"
  Signal Copy2/1 -> TargetSteerAngleCalc/9(A2)  "LCS_IN_desLaneA2"
  Signal Copy1/1 -> TargetSteerAngleCalc/8(A3)  "LCS_IN_desLaneA3"
  desLaneA0/1 -> Signal Copy5/1
  [ESS_PreDis] -> Multiport Switch4/7
  [ELK_PreDis] -> Multiport Switch4/6
  Product7/1 -> [ESS_PreDis]  "LCS_LC_ESSPredis"
  preDisMin_TB5/1 -> Product7/1, Product9/1
  Add10/1 -> Product7/2
  Constant13/1 -> Add10/1
  [DisplaySpd_kph] -> preDisMin_TB5/1, LCS_LC_ESSAES_preDis_TB/2, LCS_LC_ESSAES_preDis_TB1/2
  [Eq_A0] -> LCS_LC_ESSAES_preDis_TB/1, LCS_LC_ESSAES_preDis_TB1/1
  LCS_LC_ESSAES_preDis_TB/1 -> Add10/2  "LCS_LC_ESSPredisFac"
  LCS_LC_ELK_preDis_TB/1 -> Add9/2  "LCS_LC_ELKPredisFac"
  [Eq_A0] -> LCS_LC_ELK_preDis_TB/1, LCS_LC_ELK_preDis_TB1/1
  [DisplaySpd_kph] -> LCS_LC_ELK_preDis_TB/2, LCS_LC_ELK_preDis_TB1/2, preDisMin_TB4/1
  Constant12/1 -> Add9/1
  Add9/1 -> Product6/2
  preDisMin_TB4/1 -> Product6/1, Product8/1
  Product6/1 -> [ELK_PreDis]  "LCS_LC_ELKPredis"
  [Eq_A0] -> AngSlopeCalc/3(Eq_A0)
  Divide/1 -> [Eq_A0]  "LCS_EqA0"
  Constant7/1 -> MinMax1/2
  Constant6/1 -> MinMax/2
  MinMax/1 -> MinMax1/1
  MinMax1/1 -> Divide/2
  Constant4/1 -> Divide/3
  LaneWidth/1 -> MinMax/1
  [LCK_IE_LKA_Nomal_PreDis] -> Multiport Switch4/5
  [desLaneA0_abs] -> 2-D Lookup Table2/1
  [DisplaySpd_kph] -> 2-D Lookup Table2/2, preDisMin_TB3/1
  predis_ayFac4/1 -> Switch/1  "LCS_A2_LatAccFac"
  Constant14/1 -> Add2/1
  Add2/1 -> Product2/3
  [desLaneA2] -> Gain1/1, MATLAB Function/1(c2)
  Abs2/1 -> Product1/3
  Gain1/1 -> Abs2/1, [Curve]
  [vRef] -> Product1/2, Product1/1
  Product1/1 -> predis_ayFac4/1  "LCS_A2_LatAcc"
  preDisMin_TB3/1 -> Product2/2
  2-D Lookup Table2/1 -> Add2/2  "LCS_LCKPredisFac"
  Product2/1 -> [LCK_IE_LKA_Nomal_PreDis]  "LCS_LCKPredis"
  desLaneA0_2/1 -> AngSlopeCalc/4(desLane_A0)
  Multiport Switch4/1 -> Output2/1, [preDis]  "LCS_finalPredis"
  Direct Lookup Table (n-D)/1 -> Multiport Switch4/1  "LCS_LCType"
  AngSlopeCalc/1(AngSlope) -> Output1/1, [LCS_TarSteerAngleSlope]  "LCS_TarSteerAngleSlope"
  [Nomal_PreDis] -> Multiport Switch4/2
  [Eco_PreDis] -> Multiport Switch4/3
  [Sport_PreDis] -> Multiport Switch4/4
  Product15/1 -> [Sport_PreDis]  "LCS_LC_SportPredis"
  preDisMin_TB/1 -> Product15/1
  Add8/1 -> Product15/2
  Constant26/1 -> Add8/1
  [DisplaySpd_kph] -> preDisMin_TB/1, LCS_LC_Emergent_preDis_TB/2
  [Eq_A0] -> LCS_LC_Emergent_preDis_TB/1
  LCS_LC_Emergent_preDis_TB/1 -> Add8/2  "LCS_LC_SportPredisFac"
  Product12/1 -> [Eco_PreDis]  "LCS_LC_EcoPredis"
  LC_Medium_preDis_Fac_TB/1 -> Add7/2  "LCS_LC_EcoPredisFac"
  preDisMin_TB1/1 -> Product12/1
  [Eq_A0] -> LC_Medium_preDis_Fac_TB/1
  [DisplaySpd_kph] -> preDisMin_TB1/1, LC_Medium_preDis_Fac_TB/2
  Constant24/1 -> Add7/1
  Add7/1 -> Product12/2
  Product3/1 -> [Nomal_PreDis]  "LCS_LC_NomalPredis"
  2-D Lookup Table1/1 -> Add5/2  "LCS_LC_NomalPredisFac"
  preDisMin_TB2/1 -> Product3/1  "LCS_Predis_BaseDis"
  Add5/1 -> Product3/2
  Constant22/1 -> Add5/1
  [DisplaySpd_kph] -> preDisMin_TB2/1, 2-D Lookup Table1/2
  TarDangerlLevel2/1 -> Signal Copy6/1
  [Eq_A0] -> 2-D Lookup Table1/1
  Abs1/1 -> [desLaneA0_abs], Divide/1
  [CurrentSteerAngleOffset] -> Saturation/1
  kapTraj1/1 -> [kapTraj]
  desLaneA0_1/1 -> TargetSteerAngleCalc/11(A0)
  [DisplaySpd_kph] -> AngSlopeCalc/2(vDisplay_Kph)
  SteerAngleOffset_deg/1 -> [SteerAngleOffset_deg], Add1/2
  [SteerAngleSpd_degs] -> TargetSteerAngleCalc/13(SteerAngleSpd)
  [LineValid] -> TargetSteerAngleCalc/7(LineValid)
  Constant1/1 -> TargetSteerAngleCalc/6(R1)
  Add6/1 -> Subsystem5/1(raw), Switch1/1  "LCS_ReqEPSTrgAngle"
  canEPS_LKATorqOvrlDlvd/1 -> [canEPS_LKATorqOvrlDlvd]
  Sum/1 -> [DisplaySpd_kph]  "LCS_DisplaySpd_kph"
  Bias1/1 -> Gain5/1
  Product5/1 -> Add1/1, [LCS_IN_SteerAngle_deg]  "LCS_IN_CurSteerAngle_deg"
  canSteerWheelAngle/1 -> Product5/1
  Gain5/1 -> Product5/2
  [SteerAngle_deg] -> TargetSteerAngleCalc/3(SteerAngle)
  Add1/1 -> [SteerAngle_deg]  "LCS_CurSteerAngle_deg"
  [SteerRatio] -> TargetSteerAngleCalc/4(SteerRatio)
  Gain3/1 -> Gain4/1
  Gain4/1 -> Sum/1
  Constant8/1 -> Sum/2
  [preDis] -> TargetSteerAngleCalc/5(preDis)
  eviVxvRef_ms6/1 -> [vRef], Gain3/1
  TargetSteerAngleCalc/2(LCS_TarSteerAngleEnd) -> Terminator/1  "LCS_TarSteerAngleEnd"
  Signal Copy5/1 -> Abs1/1  "LCS_IN_desLaneA0"
  canSteerWheelAngleSign/1 -> Bias1/1
  TargetSteerAngleCalc/1(TarSteerAngle) -> Add6/1
  Constant/1 -> [SteerRatio]
  eviVxvRef_ms/1 -> TargetSteerAngleCalc/1(vRef)
  [DisplaySpd_kph] -> TargetSteerAngleCalc/2(DisplaySpd_Kph)
  desLaneA2/1 -> [desLaneA2]
  canSteerWheelSpd/1 -> Product4/1
  canSteerWheelSpdSign/1 -> Bias2/1
  Gain2/1 -> Product4/2
  Bias2/1 -> Gain2/1
  Product4/1 -> [SteerAngleSpd_degs]  "LCS_IN_SteerAngleSpd_degs"
  desLaneA3/1 -> Signal Copy1/1
  desLaneA1/1 -> Signal Copy3/1
  [desLaneA2] -> Signal Copy2/1
  TarDangerlLevel/1 -> AngSlopeCalc/1(TarDangerlLevel)
  Saturation/1 -> Add6/2
  [LCS_TarSteerAngleSlope] -> TargetSteerAngleCalc/12("TarSteerAngleSlope ")
  CurrentSteerAngleOffset/1 -> [CurrentSteerAngleOffset]
  Signal Copy/1 -> Direct Lookup Table (n-D)/1  "LCS_IN_TarDangerLevel"
  Saturation1/1 -> TargetSteerAngleCalc/14(CurrentSteerAngleOffset)
  [CurrentSteerAngleOffset] -> Saturation1/1
  [SteerAngleOffset_deg] -> Saturation2/1
  Saturation2/1 -> TargetSteerAngleCalc/15(SteerAngleOffset_deg)
  Ground1/1 -> epsTrqReqFlag/1  "LCS_OUT_EpsTrqReqValueVld"
  Ground/1 -> epsTrqReqValue/1  "LCS_OUT_EpsTrqReqValue"
  canEPS_DrvInputTorq/1 -> OverRideDetect/1(DrvTrqInput)
  Logical Operator1/1 -> [isOvride]
  OverRideDetect/1(isOverRide) -> Logical Operator1/2  "LCS_IsOverRide"
  Constant15/1 -> Logical Operator1/1
  Signal Copy4/1 -> [LineValid]  "LCS_IN_desLaneValid"
  Gain/1 -> TrgSteerAngle/1  "LCS_OUT_ReqEPSTrgAngle"

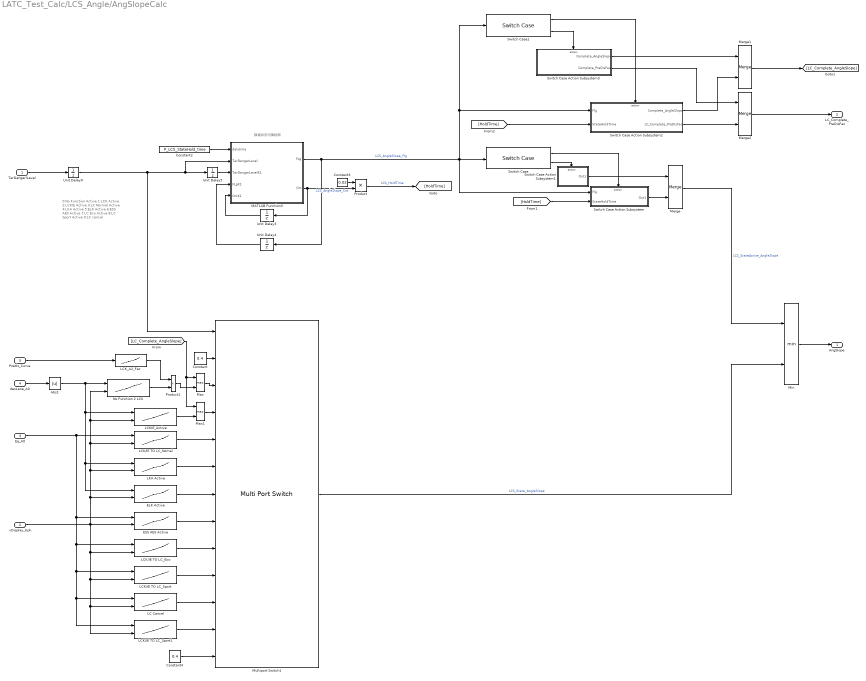
== system LATC_Test_Calc/LCS_Angle/AngSlopeCalc ==
  note: 0:No Function Active
      | 1:LCK Active
      | 2:LCKIE Active
      | 3:LC Normal Active
      | 4:LKA Active
      | 5:ELK Active
      | 6:ESS AES Active
      | 7:LC Eco Active
      | 8:LC Sport Active
      | 9:LC cancel
  note: 换道状态切换检测
  TarDangerlLevel : Inport
  vDisplay_Kph : Inport  Port=2
  Eq_A0 : Inport  Port=3
  desLane_A0 : Inport  Port=4
  Predis_Curve : Inport  Port=5
  Abs1 : Abs
  Constant : Constant  Value=0.4  OutDataTypeStr=single
  Constant2 : Constant  Value=P_LCS_StateHold_time  OutDataTypeStr=uint16
  Constant3 : Constant  Value=0.02
  Constant4 : Constant  Value=0.4  OutDataTypeStr=single
  ELK Active : Lookup_n-D  BreakpointsForDimension1=P_LCS_A0_Dis_BP  BreakpointsForDimension2=P_LCS_AngleSlope_Spd_BP  Table=P_LCS_AngleSlope_ELK  ExtrapMethod=Clip  UseLastTableValue=on  InternalRulePriority=Speed  OutDataTypeStr=single  RndMeth=Simplest
      settings: InputPortMap=u0,u1
  ESS AES Active : Lookup_n-D  BreakpointsForDimension1=P_LCS_A0_Dis_BP  BreakpointsForDimension2=P_LCS_AngleSlope_Spd_BP  Table=P_LCS_AngleSlope_ESS  ExtrapMethod=Clip  UseLastTableValue=on  InternalRulePriority=Speed  OutDataTypeStr=single  RndMeth=Simplest
      settings: InputPortMap=u0,u1
  LC Cancel : Lookup_n-D  BreakpointsForDimension1=P_LCS_A0_Dis_BP  BreakpointsForDimension2=P_LCS_AngleSlope_Spd_BP  Table=P_LCS_AngleSlope_LC_Cancel  ExtrapMethod=Clip  UseLastTableValue=on  InternalRulePriority=Speed  OutDataTypeStr=single  RndMeth=Simplest
      settings: InputPortMap=u0,u1
  LCK/IE TO LC_Eco : Lookup_n-D  BreakpointsForDimension1=P_LCS_A0_Dis_BP  BreakpointsForDimension2=P_LCS_AngleSlope_Spd_BP  Table=P_LCS_AngleSlope_LC_Eco  ExtrapMethod=Clip  UseLastTableValue=on  InternalRulePriority=Speed  OutDataTypeStr=single  RndMeth=Simplest
      settings: InputPortMap=u0,u1
  LCK/IE TO LC_Nomal : Lookup_n-D  BreakpointsForDimension1=P_LCS_A0_Dis_BP  BreakpointsForDimension2=P_LCS_AngleSlope_Spd_BP  Table=P_LCS_AngleSlope_LC_Nomal  ExtrapMethod=Clip  UseLastTableValue=on  InternalRulePriority=Speed  OutDataTypeStr=single  RndMeth=Simplest
      settings: InputPortMap=u0,u1
  LCK/IE TO LC_Sport : Lookup_n-D  BreakpointsForDimension1=P_LCS_A0_Dis_BP  BreakpointsForDimension2=P_LCS_AngleSlope_Spd_BP  Table=P_LCS_AngleSlope_LC_Sport  ExtrapMethod=Clip  UseLastTableValue=on  InternalRulePriority=Speed  OutDataTypeStr=single  RndMeth=Simplest
      settings: InputPortMap=u0,u1
  LCK/IE TO LC_Sport1 : Lookup_n-D  BreakpointsForDimension1=P_LCS_A0_Dis_BP  BreakpointsForDimension2=P_LCS_AngleSlope_Spd_BP  Table=P_LCS_AngleSlope_AES_Active  ExtrapMethod=Clip  UseLastTableValue=on  InternalRulePriority=Speed  OutDataTypeStr=single  RndMeth=Simplest
      settings: InputPortMap=u0,u1
  LCKIE_Active : Lookup_n-D  BreakpointsForDimension1=P_LCS_A0_Dis_BP  BreakpointsForDimension2=P_LCS_AngleSlope_Spd_BP  Table=P_LCS_AngleSlope_LCKIE  ExtrapMethod=Clip  UseLastTableValue=on  InternalRulePriority=Speed  OutDataTypeStr=single  RndMeth=Simplest
      settings: InputPortMap=u0,u1
  LCK_A2_Fac : Lookup_n-D  NumberOfTableDimensions=1  BreakpointsForDimension1=P_LCS_A2_Curve_BP  Table=P_LCS_AngleSlope_LCK_Curve_Fac  ExtrapMethod=Clip  UseLastTableValue=on  InternalRulePriority=Speed  RndMeth=Simplest  InputSameDT=on
  LKA Active : Lookup_n-D  BreakpointsForDimension1=P_LCS_A0_Dis_BP  BreakpointsForDimension2=P_LCS_AngleSlope_Spd_BP  Table=P_LCS_AngleSlope_LKA  ExtrapMethod=Clip  UseLastTableValue=on  InternalRulePriority=Speed  OutDataTypeStr=single  RndMeth=Simplest
      settings: InputPortMap=u0,u1
  MATLAB Function3 : MATLAB Function  TreatAsAtomicUnit=on
  Max : MinMax  Function=max  Inputs=2
  Max1 : MinMax  Function=max  Inputs=2
  Merge : Merge
  Merge1 : Merge
  Merge2 : Merge
  Min : MinMax  Inputs=2
  Multiport Switch1 : MultiPortSwitch  DataPortOrder=Zero-based contiguous  Inputs=12  zeroidx=on
  No Function 2 LCK : Lookup_n-D  BreakpointsForDimension1=P_LCS_A0_Dis_BP  BreakpointsForDimension2=P_LCS_AngleSlope_Spd_BP  Table=P_LCS_AngleSlope_LCK  ExtrapMethod=Clip  UseLastTableValue=on  InternalRulePriority=Speed  OutDataTypeStr=single  RndMeth=Simplest
      settings: InputPortMap=u0,u1
  Product : Product
  Product1 : Product
  Switch Case : SwitchCase  CaseConditions={[1,2,3,4,5,6]}
  Switch Case Action Subsystem : Subsystem  TreatAsAtomicUnit=on
  Switch Case Action Subsystem1 : Subsystem  TreatAsAtomicUnit=on
  Switch Case Action Subsystem2 : Subsystem  TreatAsAtomicUnit=on
  Switch Case Action Subsystem3 : Subsystem  TreatAsAtomicUnit=on
  Switch Case1 : SwitchCase  CaseConditions={[7,8,9,10]}
  Unit Delay{3..5,9} (4 alike) : UnitDelay  SampleTime=-1  HasFrameUpgradeWarning=on
  AngSlope : Outport  OutDataTypeStr=single
  LC_Complete_PreDisFac : Outport  Port=2  OutDataTypeStr=single
  wires:
  LCK_A2_Fac/1 -> Product1/1
  Product1/1 -> Max/2
  Predis_Curve/1 -> LCK_A2_Fac/1
  LCK/IE TO LC_Sport1/1 -> Multiport Switch1/12
  Max1/1 -> Multiport Switch1/4
  [LC_Complete_AngleSlope] -> Max/1, Max1/1
  Max/1 -> Multiport Switch1/3
  Merge2/1 -> LC_Complete_PreDisFac/1
  Merge1/1 -> [LC_Complete_AngleSlope]
  Switch Case Action Subsystem3/2(Complete_PreDisFac) -> Merge2/1
  Switch Case Action Subsystem2/2(LC_Complete_PreDisFac) -> Merge2/2
  Switch Case Action Subsystem2/1(Complete_AngleSlope) -> Merge1/2
  Switch Case Action Subsystem3/1(Complete_AngleSlope) -> Merge1/1
  Switch Case1/1 -> Switch Case Action Subsystem2/Action
  [HoldTime] -> Switch Case Action Subsystem2/2(StateHoldTime)
  Switch Case1/2 -> Switch Case Action Subsystem3/Action
  Unit Delay9/1 -> Unit Delay5/1, MATLAB Function3/2(TarDangerLevel), Multiport Switch1/1
  Eq_A0/1 -> LCK/IE TO LC_Nomal/1, ESS AES Active/1, LCK/IE TO LC_Eco/1, LCK/IE TO LC_Sport/1, LC Cancel/1, LCK/IE TO LC_Sport1/1
  Merge/1 -> Min/1  "LCS_StateActive_AngleSlope"
  Switch Case Action Subsystem1/1(Out1) -> Merge/1
  Switch Case Action Subsystem/1(Out1) -> Merge/2
  [HoldTime] -> Switch Case Action Subsystem/2(StateHoldTime)
  Switch Case/2 -> Switch Case Action Subsystem1/Action
  Switch Case/1 -> Switch Case Action Subsystem/Action
  vDisplay_Kph/1 -> ESS AES Active/2, ELK Active/2, LKA Active/2, LCK/IE TO LC_Nomal/2, LCKIE_Active/2, No Function 2 LCK/2, LCK/IE TO LC_Eco/2, LCK/IE TO LC_Sport/2, LC Cancel/2, LCK/IE TO LC_Sport1/2
  LCK/IE TO LC_Nomal/1 -> Multiport Switch1/5
  Min/1 -> AngSlope/1
  Product/1 -> [HoldTime]  "LCS_HoldTime"
  Constant3/1 -> Product/1
  desLane_A0/1 -> Abs1/1
  Constant4/1 -> Multiport Switch1/13
  LKA Active/1 -> Multiport Switch1/6
  No Function 2 LCK/1 -> Product1/2
  Multiport Switch1/1 -> Min/2  "LCS_State_AngleSlope"
  Constant2/1 -> MATLAB Function3/1(delytime)
  MATLAB Function3/1(FLg) -> Unit Delay4/1, Switch Case/1, Switch Case Action Subsystem2/1(Flg), Switch Case1/1, Switch Case Action Subsystem/1(Flg)  "LCS_AngleSlope_Flg"
  MATLAB Function3/2(Cnt) -> Unit Delay3/1, Product/2  "LCS_AngleSlope_Cnt"
  Constant/1 -> Multiport Switch1/2
  TarDangerlLevel/1 -> Unit Delay9/1
  Unit Delay4/1 -> MATLAB Function3/4(FLgK1)
  Unit Delay3/1 -> MATLAB Function3/5(CntK1)
  LCKIE_Active/1 -> Max1/2
  ELK Active/1 -> Multiport Switch1/7
  ESS AES Active/1 -> Multiport Switch1/8
  LCK/IE TO LC_Eco/1 -> Multiport Switch1/9
  LC Cancel/1 -> Multiport Switch1/11
  Abs1/1 -> No Function 2 LCK/1, LCKIE_Active/1, LKA Active/1, ELK Active/1
  LCK/IE TO LC_Sport/1 -> Multiport Switch1/10
  Unit Delay5/1 -> MATLAB Function3/3(TarDangerLevelK1)

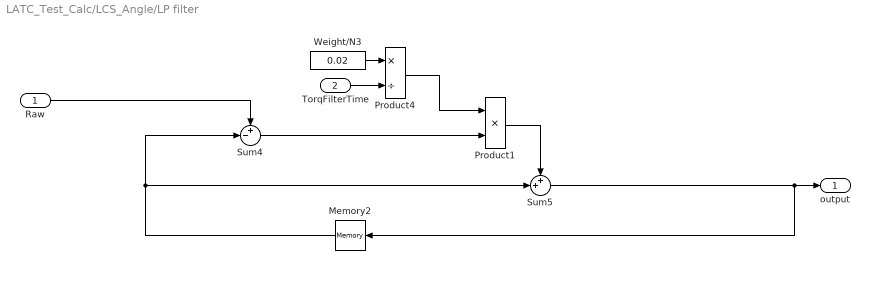
== system LATC_Test_Calc/LCS_Angle/LP filter ==
  Raw : Inport
  TorqFilterTime : Inport  Port=2
  Memory2 : Memory  InheritSampleTime=on
  Product1 : Product  RndMeth=Zero
  Product4 : Product  Inputs=*/  RndMeth=Zero
  Sum4 : Sum  Inputs=+-|
  Sum5 : Sum  Inputs=++|
  Weight/N3 : Constant  Value=0.02  OutDataTypeStr=single
  output : Outport
  wires:
  TorqFilterTime/1 -> Product4/2
  Product4/1 -> Product1/1
  Weight/N3/1 -> Product4/1
  Raw/1 -> Sum4/1
  Product1/1 -> Sum5/1
  Sum4/1 -> Product1/2
  Memory2/1 -> Sum4/2, Sum5/2
  Sum5/1 -> output/1, Memory2/1

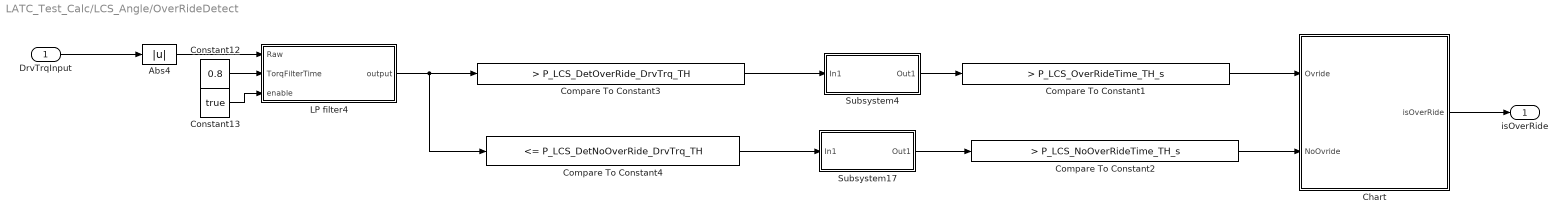
== system LATC_Test_Calc/LCS_Angle/OverRideDetect ==
  DrvTrqInput : Inport
  Abs4 : Abs
  Chart : Stateflow chart  TreatAsAtomicUnit=on
  Compare To Constant1 : simulink/Logic and Bit Operations/Compare To Constant  relop=>  const=P_LCS_OverRideTime_TH_s  OutDataTypeStr=boolean
  Compare To Constant2 : simulink/Logic and Bit Operations/Compare To Constant  relop=>  const=P_LCS_NoOverRideTime_TH_s  OutDataTypeStr=boolean
  Compare To Constant3 : simulink/Logic and Bit Operations/Compare To Constant  relop=>  const=P_LCS_DetOverRide_DrvTrq_TH  OutDataTypeStr=boolean
  Compare To Constant4 : simulink/Logic and Bit Operations/Compare To Constant  relop=<=  const=P_LCS_DetNoOverRide_DrvTrq_TH  OutDataTypeStr=boolean
  Constant12 : Constant  Value=0.8
  Constant13 : Constant  Value=true
  LP filter4 : Subsystem
  Subsystem17 : Subsystem  mask{Ts=0.02, Max=10}
      mask prompts: Ts "Sample Time:"; Max "Max Limit:"
      mask Display:
      | Ts=get_param(gcb,'Ts');
      | Max=get_param(gcb,'Max');
      | disp(['Ts:' Ts '\n' 'Max:' Max ]);
  Subsystem4 : Subsystem  mask{Ts=0.02, Max=10}
      mask prompts: Ts "Sample Time:"; Max "Max Limit:"
      mask Display:
      | Ts=get_param(gcb,'Ts');
      | Max=get_param(gcb,'Max');
      | disp(['Ts:' Ts '\n' 'Max:' Max ]);
  isOverRide : Outport
  wires:
  Compare To Constant2/1 -> Chart/2(NoOvride)
  Compare To Constant1/1 -> Chart/1(Ovride)
  DrvTrqInput/1 -> Abs4/1
  Constant13/1 -> LP filter4/3(enable)
  Compare To Constant3/1 -> Subsystem4/1(In1)
  LP filter4/1(output) -> Compare To Constant3/1, Compare To Constant4/1
  Chart/1(isOverRide) -> isOverRide/1
  Constant12/1 -> LP filter4/2(TorqFilterTime)
  Abs4/1 -> LP filter4/1(Raw)
  Subsystem4/1(Out1) -> Compare To Constant1/1
  Subsystem17/1(Out1) -> Compare To Constant2/1
  Compare To Constant4/1 -> Subsystem17/1(In1)

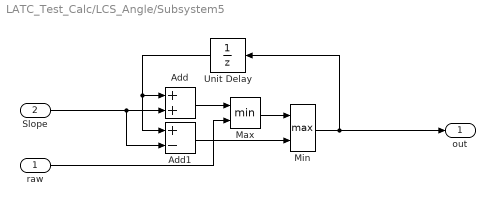
== system LATC_Test_Calc/LCS_Angle/Subsystem5 ==
  raw : Inport
  Slope : Inport  Port=2
  Add : Sum
  Add1 : Sum  Inputs=+-
  Max : MinMax  Inputs=2
  Min : MinMax  Function=max  Inputs=2
  Unit Delay : UnitDelay  InitialCondition=single(0)  SampleTime=-1  HasFrameUpgradeWarning=on
  out : Outport
  wires:
  Slope/1 -> Add1/2, Add/2
  Unit Delay/1 -> Add1/1, Add/1
  Min/1 -> out/1, Unit Delay/1
  Max/1 -> Min/1
  Add/1 -> Max/1
  Add1/1 -> Min/2
  raw/1 -> Max/2
